simulink model "Power_Grid_Fault_Analysis_2016"  (R2016a)
settings: Solver=FixedStepAuto  SolverMode=SingleTasking  StartTime=0.0  StopTime=0.2  RelTol=1e-3
InitFcn:
  | basekV = 23;
  | baseMVA = 100;
  | 
  | % base impedance
  | baseZ = (basekV)^2/baseMVA;
  | 
  | % nominal frequency
  | freq = 50;
libraries: powerlib x64, powerlib_meascontrol x17
(part 4 of 4)

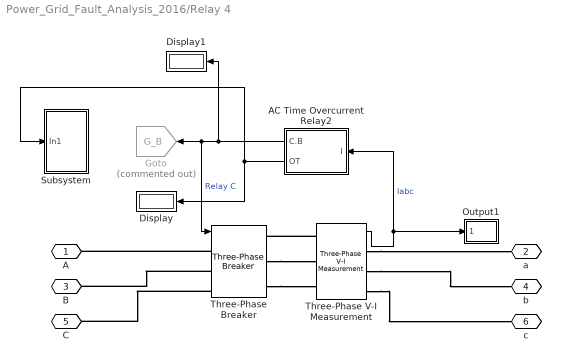
== system Power_Grid_Fault_Analysis_2016/Relay 4 ==
  AC Time Overcurrent Relay2 : Subsystem  mask(AC Time Overcurrent Relay Block){tcpopup=Definite Minimum Time, k=0, alpha=0.02, B=0, PS=100%, TMS=0.1, TDS=5, CTpri=300, CTsec=5, Freq=60, RMSInit=0}
      mask prompts: tcpopup "Trip Characteristic"; PS "Plug Setting (PS) / Low-set (I >)"; TMS "Time Multiplier Setting (TMS)"; TDS "Time Delay Setting (TDS) in sec"; CTpri "Current Transformer Primary (A)"; CTsec "Current Transformer Secondary (A)"; Freq "Fundamental frequency (Hz):"; RMSInit "Initial RMS value:"
      mask help:
      | AC Time Overcurrent Relay Block developed by Dr Rodney Tan
      | Version 1.0 (Jun 2016)
      |
      | AC Time Overcurrent Relay (ANSI/IEEE C37.2 device number 51) that operates when the current exceeds a predetermined value.
      |
      | This relay operates with either a Definite Minimum Time (DMT) or Inverse Definite Minimum Time (IDMT) characteristic.
      |
      | This relay support both IEC 60255 Standard and IEEE Standard C37.112-1996 IDMT trip characteristic.
      mask Help:
      | <b><u>Block Setting</u></b>
      | <b>Trip Characteristic</b>
      | Relay operation mode selection of Definite Minimum Time (DMT), IEC 60255 Standard or IEEE Standard C37.112-1996 Inverse Definite Minimum Time (IDMT).
      | 
      | <b>Plug-Setting(PS) / Low-set (I >)</b>
      | Specify relay pick-up current based on current transformer rating ranging from 25% to 200% with 25% step interval.
      | 
      | <b>Time Multiplier Setting (TMS)</b>
      | Specify time delay multiplier ranging from 0.05 to 1.0 for IDMT relay operation. This setting will be disabled DMT relay operation mode.
      | 
      | <b>Plot Curve Button</b>
      | Plot current Inverse Definite Minimum Time trip curve.
      | 
      | <b>Time Delay Setting (TDS)</b>
      | Specify time delay ranging from 0.05sec to 99sec for Definite Minimum Time relay operation. This setting will be disabled in IDMT relay operation mode.
      | 
      | <b>Current Transformer Primary (A)</b>
      | Specify current transformer primary in Ampere.
      | 
      | <b>Current Transformer Secondary (A)</b>
      | Specify current transformer secondary in Ampere.
      | 
      | <b>Fundamental Frequency (Hz)</b>
      | Specify the RMS current measurement fundamental frequency, in hertz, of the input signal.
      | 
      | <b>Initial RMS Value</b>
      | Specify the RMS current measurement initial RMS value of the output signal.
      | 
      | <b><u>Block Input Output</u></b>
      | <b>I</b>
      | Current input to the AC time overcurrent relay
      | 
      | <b>trip</b>
      | Trip control signal output (1-0), commonly connected to circuit breaker
      | 
      | <b>OT</b>
      | Relay operating time output
      mask TypeOptions tcpopup: Definite Minimum Time | IEC Standard Inverse | IEC Very Inverse | IEC Long Time Inverse | IEC Extremely Inverse | IEC Ultra Inverse | IEEE Moderately Inverse | IEEE Very Inverse | IEEE Extremely Inverse
      mask Callback tcpopup:
      | switch(get_param(gcb,'tcpopup'))
      |     case 'IEC Standard Inverse'
      |         set_param(gcb,'k','0.14');
      |         set_param(gcb,'alpha','0.02');
      |         set_param(gcb,'B','0');
      |         set_param(gcb,'MaskEnables',{'on','off','off','off',...
      |                   'on','on','off','on','on','on','on'});
      |     case 'IEC Very Inverse'
      |         set_param(gcb,'k','13.5');
      |         set_param(gcb,'alpha','1');
      |         set_param(gcb,'B','0');
      |         set_param(gcb,'MaskEnables',{'on','off','off','off',...
      |                   'on','on','off','on','on','on','on'});
      |     case 'IEC Long Time Inverse'
      |         set_param(gcb,'k','120');
      |         set_param(gcb,'alpha','1');
      |         set_param(gcb,'B','0');
      |         set_param(gcb,'MaskEnables',{'on','off','off','off',...
      |                   'on','on','off','on','on','on','on'});
      |     case 'IEC Extremely Inverse'
      |         set_param(gcb,'k','80');
      |         set_param(gcb,'alpha','2');
      |         set_param(gcb,'B','0');
      |         set_param(gcb,'MaskEnables',{'on','off','off','off',...
      |                   'on','on','off','on','on','on','on'});
      |     case 'IEC Ultra Inverse'
      |         set_param(gcb,'k','315.2');
      |         set_param(gcb,'alpha','2.5');
      |         set_param(gcb,'B','0');
      |         set_param(gcb,'MaskEnables',{'on','off','off','off',...
      |                   'on','on','off','on','on','on','on'});
      |     case 'IEEE Moderately Inverse'
      |         set_param(gcb,'k','0.0515');
      |         set_param(gcb,'alpha','0.02');
      |         set_param(gcb,'B','0.114');
      |         set_param(gcb,'MaskEnables',{'on','off','off','off',...
      |                   'on','on','off','on','on','on','on'});
      |     case 'IEEE Very Inverse'
      |         set_param(gcb,'k','19.61');
      |         set_param(gcb,'alpha','2');
      |         set_param(gcb,'B','0.491');
      |         set_param(gcb,'MaskEnables',{'on','off','off','off',...
      |                   'on','on','off','on','on','on','on'});
      |     case 'IEEE Extremely Inverse'
      |         set_param(gcb,'k','28.2');
      |         set_param(gcb,'alpha','2');
      |         set_param(gcb,'B','0.1217');
      |         set_param(gcb,'MaskEnables',{'on','off','off','off',...
      |                   'on','on','off','on','on','on','on'});
      |     otherwise
      |         set_param(gcb,'k','0');
      |         set_param(gcb,'MaskEnables',{'on','off','off','off',...
      |                   'on','off','on','on','on','on','on'});
      | end
      mask TypeOptions PS: 25% | 50% | 75% | 100% | 125% | 150% | 175% | 200%
      mask TypeOptions TMS: 0.05 | 0.1 | 0.15 | 0.2 | 0.25 | 0.3 | 0.35 | 0.4 | 0.45 | 0.5 | 0.55 | 0.6 | 0.65 | 0.7 | 0.75 | 0.8 | 0.85 | 0.9 | 0.95 | 1.0
      mask Callback TDS:
      | TDS = str2double(get_param(gcb,'TDS'));
      | if (TDS > 99)||(TDS < 0.05)||isnan(TDS)
      |     msgbox('TDS must be in the range of 0.05-99 sec',...
      |     'Invalid Value !','error');
      |     set_param(gcb,'TDS','0.1');
      | end
      mask TypeOptions Freq: Irms/Freq
      mask TypeOptions RMSInit: Irms/RMSInit
      mask DialogControl plotbutton Prompt: Plot Curve
      mask DialogControl plotbutton Callback:
      | % Plotting IDMT Curve
      | TMS = str2num(get_param(gcb,'TMS'));
      | k = str2num(get_param(gcb,'k'));
      | alpha = str2num(get_param(gcb,'alpha'));
      | B = str2num(get_param(gcb,'B'));
      | I = 1:20;
      | td = ((k./((I.^alpha)-1))+B)*TMS;
      | loglog(td);
      | set(gcf, 'Position', [200 150 300 500]);
      | switch(get_param(gcb,'tcpopup'))
      |     case 'IEC Standard Inverse'
      |         title('IEC Standard Inverse');
      |         set(gca, 'YTick', (1:10));
      |         ylim([0.1 10]);
      |     case 'IEC Very Inverse'
      |         title('IEC Very Inverse');
      |         set(gca, 'YTick', (1:2:15));
      |         ylim([0.01 15]);
      |     case 'IEC Long Time Inverse'
      |         title('IEC Long Time Inverse');
      |         set(gca, 'YTick', (0:20:120));
      |         ylim([0.1 120]);
      |     case 'IEC Extremely Inverse'
      |         title('IEC Extremely Inverse');
      |         set(gca, 'YTick', (0:5:30));
      |         ylim([0.01 30]);
      |     case 'IEC Ultra Inverse'
      |         title('IEC Ultra Inverse');
      |         set(gca, 'YTick', (0:20:100));
      |         ylim([0.01 100]);
      |     case 'IEEE Moderately Inverse'
      |         title('IEEE Moderately Inverse');
      |         set(gca, 'YTick', (1:5));
      |         ylim([0.01 5]);
      |     case 'IEEE Very Inverse'
      |         title('IEEE Very Inverse');
      |         set(gca, 'YTick', (1:10));
      |         ylim([0.01 10]);
      |     case 'IEEE Extremely Inverse'
      |         title('IEEE Extremely Inverse');
      |         set(gca, 'YTick', (1:10));
      |         ylim([0.01 10]);
      | end
      | 
      | set(gca, 'XTick', [1:10 20]);
      | xlim([1 30]);
      | xlabel('Current (Multiples of Plug Setting)');
      | ylabel('Operating Time (sec)');
      | grid on;
      mask DialogControl RMS Prompt: RMS Current Measurement
      mask Display:
      | disp('(51)');
      | port_label('input', 1, 'I');
      | port_label('output', 1, 'trip');
      | port_label('output', 2, 'OT');
  Display : Display
  Display1 : Display
  Goto : Goto  Commented=on  GotoTag=G_B  TagVisibility=global
  Output1 : Subsystem
  Subsystem : Subsystem
  Three-Phase V-I Measurement : powerlib/Measurements/Three-Phase V-I Measurement  VoltageMeasurement=no  SetLabelV=off  LabelV=Vabc  Vpu=off  VpuLL=off  CurrentMeasurement=yes  SetLabelI=off  LabelI=Iabc  Ipu=off  Pbase=100e6  Vbase=500e3  OutputType=Complex  PhasorSimulation=off  PSBequivalent=0
  Three-Phase Breaker : powerlib/Elements/Three-Phase Breaker  InitialState=closed  SwitchA=on  SwitchB=on  SwitchC=on  SwitchTimes="[1/60  5/60]"  External=on  BreakerResistance=0.001  SnubberResistance=1e6  SnubberCapacitance=inf  Measurements=None
  A : PMIOPort  Side=Left
  a : PMIOPort  Port=2  Side=Right
  B : PMIOPort  Port=3  Side=Left
  b : PMIOPort  Port=4  Side=Right
  C : PMIOPort  Port=5  Side=Left
  c : PMIOPort  Port=6  Side=Right
  wires:
  Three-Phase V-I Measurement/1 -> Output1/1(Signal), AC Time Overcurrent Relay2/1(I)  "Iabc"
  AC Time Overcurrent Relay2/2(OT) -> Subsystem/1(In1), Display/1
  AC Time Overcurrent Relay2/1(C.B) -> Display1/1, Goto/1, Three-Phase Breaker/1  "Relay C"
  connections:
  Three-Phase Breaker/RConn2 -- Three-Phase V-I Measurement/LConn2
  Three-Phase V-I Measurement/RConn2 -- b/RConn1
  Three-Phase V-I Measurement/LConn1 -- Three-Phase Breaker/RConn1
  Three-Phase Breaker/LConn2 -- B/RConn1
  Three-Phase V-I Measurement/RConn1 -- a/RConn1
  Three-Phase Breaker/RConn3 -- Three-Phase V-I Measurement/LConn3
  Three-Phase Breaker/LConn3 -- C/RConn1
  Three-Phase V-I Measurement/RConn3 -- c/RConn1
  Three-Phase Breaker/LConn1 -- A/RConn1

== system Power_Grid_Fault_Analysis_2016/Toggle Switch ==

== system Power_Grid_Fault_Analysis_2016/Toggle Switch1 ==

== system Power_Grid_Fault_Analysis_2016/Toggle Switch2 ==

== system Power_Grid_Fault_Analysis_2016/Toggle Switch3 ==

== system Power_Grid_Fault_Analysis_2016/Toggle Switch4 ==

== system Power_Grid_Fault_Analysis_2016/Bus_10/VI Recorder7 ==
  Vrec : Inport
  Irec : Inport  Port=2
  tag scope: I8to10=global, V8to10=global
  wires:
  Vrec/1 -> [V8to10]
  Irec/1 -> [I8to10]

== system Power_Grid_Fault_Analysis_2016/Bus_11/VI Recorder7 ==
  Vrec : Inport
  Irec : Inport  Port=2
  tag scope: I9to11=global, V9to11=global
  wires:
  Vrec/1 -> [V9to11]
  Irec/1 -> [I9to11]

== system Power_Grid_Fault_Analysis_2016/Bus_12/VI Recorder7 ==
  Vrec : Inport
  Irec : Inport  Port=2
  tag scope: I9to12=global, V9to12=global
  wires:
  Vrec/1 -> [V9to12]
  Irec/1 -> [I9to12]

== system Power_Grid_Fault_Analysis_2016/Bus_13/VI Recorder7 ==
  Vrec : Inport
  Irec : Inport  Port=2
  tag scope: I3to13=global, V3to13=global
  wires:
  Vrec/1 -> [V3to13]
  Irec/1 -> [I3to13]

== system Power_Grid_Fault_Analysis_2016/Bus_14/VI Recorder7 ==
  Vrec : Inport
  Irec : Inport  Port=2
  tag scope: I13to14=global, V13to14=global
  wires:
  Vrec/1 -> [V13to14]
  Irec/1 -> [I13to14]

== system Power_Grid_Fault_Analysis_2016/Bus_15/VI Recorder7 ==
  Vrec : Inport
  Irec : Inport  Port=2
  tag scope: I13to15=global, V13to15=global
  wires:
  Vrec/1 -> [V13to15]
  Irec/1 -> [I13to15]

== system Power_Grid_Fault_Analysis_2016/Bus_16/VI Recorder7 ==
  Vrec : Inport
  Irec : Inport  Port=2
  tag scope: I15to16=global, V15to16=global
  wires:
  Vrec/1 -> [V15to16]
  Irec/1 -> [I15to16]

== system Power_Grid_Fault_Analysis_2016/Bus_4/VI Recorder7 ==
  Vrec : Inport
  Irec : Inport  Port=2
  tag scope: I1to4=global, V1to4=global
  wires:
  Vrec/1 -> [V1to4]
  Irec/1 -> [I1to4]

== system Power_Grid_Fault_Analysis_2016/Bus_5/VI Recorder7 ==
  Vrec : Inport
  Irec : Inport  Port=2
  tag scope: I4to5=global, V4to5=global
  wires:
  Vrec/1 -> [V4to5]
  Irec/1 -> [I4to5]

== system Power_Grid_Fault_Analysis_2016/Bus_6/VI Recorder7 ==
  Vrec : Inport
  Irec : Inport  Port=2
  tag scope: I4to6=global, V4to6=global
  wires:
  Vrec/1 -> [V4to6]
  Irec/1 -> [I4to6]

== system Power_Grid_Fault_Analysis_2016/Bus_7/VI Recorder7 ==
  Vrec : Inport
  Irec : Inport  Port=2
  tag scope: I6to7=global, V6to7=global
  wires:
  Vrec/1 -> [V6to7]
  Irec/1 -> [I6to7]

== system Power_Grid_Fault_Analysis_2016/Bus_8/VI Recorder7 ==
  Vrec : Inport
  Irec : Inport  Port=2
  tag scope: I2to8=global, V2to8=global
  wires:
  Vrec/1 -> [V2to8]
  Irec/1 -> [I2to8]

== system Power_Grid_Fault_Analysis_2016/Bus_9/VI Recorder7 ==
  Vrec : Inport
  Irec : Inport  Port=2
  tag scope: I8to9=global, V8to9=global
  wires:
  Vrec/1 -> [V8to9]
  Irec/1 -> [I8to9]

== system Power_Grid_Fault_Analysis_2016/For Zone 1/If Action Subsystem ==
  Input : Inport
  Input1 : Inport  Port=2
  Input2 : Inport  Port=3
  Action Port : ActionPort
  Out1 : Outport
  Out2 : Outport  Port=2
  Out3 : Outport  Port=3
  wires:
  Input/1 -> Out1/1
  Input1/1 -> Out2/1
  Input2/1 -> Out3/1

== system Power_Grid_Fault_Analysis_2016/For Zone 1/If Action Subsystem1 ==
  Input : Inport
  Input1 : Inport  Port=2
  Input2 : Inport  Port=3
  Action Port : ActionPort
  Out1 : Outport
  Out2 : Outport  Port=2
  Out3 : Outport  Port=3
  wires:
  Input/1 -> Out1/1
  Input1/1 -> Out2/1
  Input2/1 -> Out3/1

== system Power_Grid_Fault_Analysis_2016/For Zone 1/If Action Subsystem2 ==
  Input : Inport
  Input1 : Inport  Port=2
  Input2 : Inport  Port=3
  Action Port : ActionPort
  Out1 : Outport
  Out2 : Outport  Port=2
  Out3 : Outport  Port=3
  wires:
  Input/1 -> Out1/1
  Input1/1 -> Out2/1
  Input2/1 -> Out3/1

== system Power_Grid_Fault_Analysis_2016/For Zone 1/If Action Subsystem3 ==
  Input : Inport
  Input1 : Inport  Port=2
  Input2 : Inport  Port=3
  Action Port : ActionPort
  Out1 : Outport
  Out2 : Outport  Port=2
  Out3 : Outport  Port=3
  wires:
  Input/1 -> Out1/1
  Input1/1 -> Out2/1
  Input2/1 -> Out3/1

== system Power_Grid_Fault_Analysis_2016/For Zone 1/If Action Subsystem4 ==
  Input : Inport
  Input1 : Inport  Port=2
  Input2 : Inport  Port=3
  Action Port : ActionPort
  Out1 : Outport
  Out2 : Outport  Port=2
  Out3 : Outport  Port=3
  wires:
  Input/1 -> Out1/1
  Input1/1 -> Out2/1
  Input2/1 -> Out3/1

== system Power_Grid_Fault_Analysis_2016/For Zone 1/If Action Subsystem5 ==
  Input : Inport
  Input1 : Inport  Port=2
  Input2 : Inport  Port=3
  Action Port : ActionPort
  Out1 : Outport
  Out2 : Outport  Port=2
  Out3 : Outport  Port=3
  wires:
  Input/1 -> Out1/1
  Input1/1 -> Out2/1
  Input2/1 -> Out3/1

== system Power_Grid_Fault_Analysis_2016/For Zone 1/If Action Subsystem6 ==
  Input : Inport
  Input1 : Inport  Port=2
  Input2 : Inport  Port=3
  Action Port : ActionPort
  Out1 : Outport
  Out2 : Outport  Port=2
  Out3 : Outport  Port=3
  wires:
  Input/1 -> Out1/1
  Input1/1 -> Out2/1
  Input2/1 -> Out3/1

== system Power_Grid_Fault_Analysis_2016/For Zone 1/Subsystem1 ==
  In1 : Inport
  In2 : Inport  Port=2
  Display2 : Display
      settings: Decimation=2
  Divide4 : Product  Inputs=**  SaturateOnIntegerOverflow=on  RndMeth=Zero
  Output : Outport
  wires:
  Divide4/1 -> Display2/1, Output/1
  In1/1 -> Divide4/1
  In2/1 -> Divide4/2

== system Power_Grid_Fault_Analysis_2016/For Zone 1/Subsystem2 ==
  In1 : Inport
  In2 : Inport  Port=2
  Display2 : Display
      settings: Decimation=2
  Divide4 : Product  Inputs=**  SaturateOnIntegerOverflow=on  RndMeth=Zero
  Output : Outport
  wires:
  In2/1 -> Divide4/2
  In1/1 -> Divide4/1
  Divide4/1 -> Output/1, Display2/1

== system Power_Grid_Fault_Analysis_2016/For Zone 1/Subsystem3 ==
  In1 : Inport
  In2 : Inport  Port=2
  Display2 : Display
      settings: Decimation=2
  Divide4 : Product  Inputs=**  SaturateOnIntegerOverflow=on  RndMeth=Zero
  Output : Outport
  wires:
  In2/1 -> Divide4/2
  In1/1 -> Divide4/1
  Divide4/1 -> Output/1, Display2/1

== system Power_Grid_Fault_Analysis_2016/For Zone 1/Subsystem4 ==
  In1 : Inport
  In2 : Inport  Port=2
  Display2 : Display
      settings: Decimation=2
  Divide4 : Product  Inputs=**  SaturateOnIntegerOverflow=on  RndMeth=Zero
  Output : Outport
  wires:
  Divide4/1 -> Display2/1, Output/1
  In1/1 -> Divide4/1
  In2/1 -> Divide4/2

== system Power_Grid_Fault_Analysis_2016/For Zone 1/Subsystem5 ==
  In1 : Inport
  In2 : Inport  Port=2
  Display2 : Display
      settings: Decimation=2
  Divide4 : Product  Inputs=**  SaturateOnIntegerOverflow=on  RndMeth=Zero
  Output : Outport
  wires:
  In2/1 -> Divide4/2
  In1/1 -> Divide4/1
  Divide4/1 -> Output/1, Display2/1

== system Power_Grid_Fault_Analysis_2016/For Zone 1/Subsystem6 ==
  In1 : Inport
  In2 : Inport  Port=2
  Display2 : Display
      settings: Decimation=2
  Divide4 : Product  Inputs=**  SaturateOnIntegerOverflow=on  RndMeth=Zero
  Output : Outport
  wires:
  Divide4/1 -> Display2/1, Output/1
  In1/1 -> Divide4/1
  In2/1 -> Divide4/2

== system Power_Grid_Fault_Analysis_2016/For Zone 1/Subsystem7 ==
  In1 : Inport
  In2 : Inport  Port=2
  Display2 : Display
      settings: Decimation=2
  Divide4 : Product  Inputs=**  SaturateOnIntegerOverflow=on  RndMeth=Zero
  Output : Outport
  wires:
  In2/1 -> Divide4/2
  In1/1 -> Divide4/1
  Divide4/1 -> Output/1, Display2/1

== system Power_Grid_Fault_Analysis_2016/For Zone 2/If Action Subsystem ==
  Input : Inport
  Input1 : Inport  Port=2
  Input2 : Inport  Port=3
  Action Port : ActionPort
  Out1 : Outport
  Out2 : Outport  Port=2
  Out3 : Outport  Port=3
  wires:
  Input/1 -> Out1/1
  Input1/1 -> Out2/1
  Input2/1 -> Out3/1

== system Power_Grid_Fault_Analysis_2016/For Zone 2/If Action Subsystem1 ==
  Input : Inport
  Input1 : Inport  Port=2
  Input2 : Inport  Port=3
  Action Port : ActionPort
  Out1 : Outport
  Out2 : Outport  Port=2
  Out3 : Outport  Port=3
  wires:
  Input/1 -> Out1/1
  Input1/1 -> Out2/1
  Input2/1 -> Out3/1

== system Power_Grid_Fault_Analysis_2016/For Zone 2/If Action Subsystem2 ==
  Input : Inport
  Input1 : Inport  Port=2
  Input2 : Inport  Port=3
  Action Port : ActionPort
  Out1 : Outport
  Out2 : Outport  Port=2
  Out3 : Outport  Port=3
  wires:
  Input/1 -> Out1/1
  Input1/1 -> Out2/1
  Input2/1 -> Out3/1

== system Power_Grid_Fault_Analysis_2016/For Zone 2/If Action Subsystem3 ==
  Input : Inport
  Input1 : Inport  Port=2
  Input2 : Inport  Port=3
  Action Port : ActionPort
  Out1 : Outport
  Out2 : Outport  Port=2
  Out3 : Outport  Port=3
  wires:
  Input/1 -> Out1/1
  Input1/1 -> Out2/1
  Input2/1 -> Out3/1

== system Power_Grid_Fault_Analysis_2016/For Zone 2/If Action Subsystem4 ==
  Input : Inport
  Input1 : Inport  Port=2
  Input2 : Inport  Port=3
  Action Port : ActionPort
  Out1 : Outport
  Out2 : Outport  Port=2
  Out3 : Outport  Port=3
  wires:
  Input/1 -> Out1/1
  Input1/1 -> Out2/1
  Input2/1 -> Out3/1

== system Power_Grid_Fault_Analysis_2016/For Zone 2/If Action Subsystem5 ==
  Input : Inport
  Input1 : Inport  Port=2
  Input2 : Inport  Port=3
  Action Port : ActionPort
  Out1 : Outport
  Out2 : Outport  Port=2
  Out3 : Outport  Port=3
  wires:
  Input/1 -> Out1/1
  Input1/1 -> Out2/1
  Input2/1 -> Out3/1

== system Power_Grid_Fault_Analysis_2016/For Zone 2/If Action Subsystem6 ==
  Input : Inport
  Input1 : Inport  Port=2
  Input2 : Inport  Port=3
  Action Port : ActionPort
  Out1 : Outport
  Out2 : Outport  Port=2
  Out3 : Outport  Port=3
  wires:
  Input/1 -> Out1/1
  Input1/1 -> Out2/1
  Input2/1 -> Out3/1

== system Power_Grid_Fault_Analysis_2016/For Zone 2/Subsystem1 ==
  In1 : Inport
  In2 : Inport  Port=2
  Display2 : Display
      settings: Decimation=2
  Divide4 : Product  Inputs=**  SaturateOnIntegerOverflow=on  RndMeth=Zero
  Output : Outport
  wires:
  Divide4/1 -> Display2/1, Output/1
  In1/1 -> Divide4/1
  In2/1 -> Divide4/2

== system Power_Grid_Fault_Analysis_2016/For Zone 2/Subsystem2 ==
  In1 : Inport
  In2 : Inport  Port=2
  Display2 : Display
      settings: Decimation=2
  Divide4 : Product  Inputs=**  SaturateOnIntegerOverflow=on  RndMeth=Zero
  Output : Outport
  wires:
  In2/1 -> Divide4/2
  In1/1 -> Divide4/1
  Divide4/1 -> Output/1, Display2/1

== system Power_Grid_Fault_Analysis_2016/For Zone 2/Subsystem3 ==
  In1 : Inport
  In2 : Inport  Port=2
  Display2 : Display
      settings: Decimation=2
  Divide4 : Product  Inputs=**  SaturateOnIntegerOverflow=on  RndMeth=Zero
  Output : Outport
  wires:
  In2/1 -> Divide4/2
  In1/1 -> Divide4/1
  Divide4/1 -> Output/1, Display2/1

== system Power_Grid_Fault_Analysis_2016/For Zone 2/Subsystem4 ==
  In1 : Inport
  In2 : Inport  Port=2
  Display2 : Display
      settings: Decimation=2
  Divide4 : Product  Inputs=**  SaturateOnIntegerOverflow=on  RndMeth=Zero
  Output : Outport
  wires:
  Divide4/1 -> Display2/1, Output/1
  In1/1 -> Divide4/1
  In2/1 -> Divide4/2

== system Power_Grid_Fault_Analysis_2016/For Zone 2/Subsystem5 ==
  In1 : Inport
  In2 : Inport  Port=2
  Display2 : Display
      settings: Decimation=2
  Divide4 : Product  Inputs=**  SaturateOnIntegerOverflow=on  RndMeth=Zero
  Output : Outport
  wires:
  In2/1 -> Divide4/2
  In1/1 -> Divide4/1
  Divide4/1 -> Output/1, Display2/1

== system Power_Grid_Fault_Analysis_2016/For Zone 2/Subsystem6 ==
  In1 : Inport
  In2 : Inport  Port=2
  Display2 : Display
      settings: Decimation=2
  Divide4 : Product  Inputs=**  SaturateOnIntegerOverflow=on  RndMeth=Zero
  Output : Outport
  wires:
  Divide4/1 -> Display2/1, Output/1
  In1/1 -> Divide4/1
  In2/1 -> Divide4/2

== system Power_Grid_Fault_Analysis_2016/For Zone 2/Subsystem7 ==
  In1 : Inport
  In2 : Inport  Port=2
  Display2 : Display
      settings: Decimation=2
  Divide4 : Product  Inputs=**  SaturateOnIntegerOverflow=on  RndMeth=Zero
  Output : Outport
  wires:
  In2/1 -> Divide4/2
  In1/1 -> Divide4/1
  Divide4/1 -> Output/1, Display2/1

== system Power_Grid_Fault_Analysis_2016/For Zone 3/If Action Subsystem ==
  Input : Inport
  Input1 : Inport  Port=2
  Input2 : Inport  Port=3
  Action Port : ActionPort
  Out1 : Outport
  Out2 : Outport  Port=2
  Out3 : Outport  Port=3
  wires:
  Input/1 -> Out1/1
  Input1/1 -> Out2/1
  Input2/1 -> Out3/1

== system Power_Grid_Fault_Analysis_2016/For Zone 3/If Action Subsystem1 ==
  Input : Inport
  Input1 : Inport  Port=2
  Input2 : Inport  Port=3
  Action Port : ActionPort
  Out1 : Outport
  Out2 : Outport  Port=2
  Out3 : Outport  Port=3
  wires:
  Input/1 -> Out1/1
  Input1/1 -> Out2/1
  Input2/1 -> Out3/1

== system Power_Grid_Fault_Analysis_2016/For Zone 3/If Action Subsystem2 ==
  Input : Inport
  Input1 : Inport  Port=2
  Input2 : Inport  Port=3
  Action Port : ActionPort
  Out1 : Outport
  Out2 : Outport  Port=2
  Out3 : Outport  Port=3
  wires:
  Input/1 -> Out1/1
  Input1/1 -> Out2/1
  Input2/1 -> Out3/1

== system Power_Grid_Fault_Analysis_2016/For Zone 3/If Action Subsystem3 ==
  Input : Inport
  Input1 : Inport  Port=2
  Input2 : Inport  Port=3
  Action Port : ActionPort
  Out1 : Outport
  Out2 : Outport  Port=2
  Out3 : Outport  Port=3
  wires:
  Input/1 -> Out1/1
  Input1/1 -> Out2/1
  Input2/1 -> Out3/1

== system Power_Grid_Fault_Analysis_2016/For Zone 3/If Action Subsystem4 ==
  Input : Inport
  Input1 : Inport  Port=2
  Input2 : Inport  Port=3
  Action Port : ActionPort
  Out1 : Outport
  Out2 : Outport  Port=2
  Out3 : Outport  Port=3
  wires:
  Input/1 -> Out1/1
  Input1/1 -> Out2/1
  Input2/1 -> Out3/1

== system Power_Grid_Fault_Analysis_2016/For Zone 3/If Action Subsystem5 ==
  Input : Inport
  Input1 : Inport  Port=2
  Input2 : Inport  Port=3
  Action Port : ActionPort
  Out1 : Outport
  Out2 : Outport  Port=2
  Out3 : Outport  Port=3
  wires:
  Input/1 -> Out1/1
  Input1/1 -> Out2/1
  Input2/1 -> Out3/1

== system Power_Grid_Fault_Analysis_2016/For Zone 3/If Action Subsystem6 ==
  Input : Inport
  Input1 : Inport  Port=2
  Input2 : Inport  Port=3
  Action Port : ActionPort
  Out1 : Outport
  Out2 : Outport  Port=2
  Out3 : Outport  Port=3
  wires:
  Input/1 -> Out1/1
  Input1/1 -> Out2/1
  Input2/1 -> Out3/1

== system Power_Grid_Fault_Analysis_2016/For Zone 3/Subsystem1 ==
  In1 : Inport
  In2 : Inport  Port=2
  Display2 : Display
      settings: Decimation=2
  Divide4 : Product  Inputs=**  SaturateOnIntegerOverflow=on  RndMeth=Zero
  Output : Outport
  wires:
  Divide4/1 -> Display2/1, Output/1
  In1/1 -> Divide4/1
  In2/1 -> Divide4/2

== system Power_Grid_Fault_Analysis_2016/For Zone 3/Subsystem2 ==
  In1 : Inport
  In2 : Inport  Port=2
  Display2 : Display
      settings: Decimation=2
  Divide4 : Product  Inputs=**  SaturateOnIntegerOverflow=on  RndMeth=Zero
  Output : Outport
  wires:
  In2/1 -> Divide4/2
  In1/1 -> Divide4/1
  Divide4/1 -> Output/1, Display2/1

== system Power_Grid_Fault_Analysis_2016/For Zone 3/Subsystem3 ==
  In1 : Inport
  In2 : Inport  Port=2
  Display2 : Display
      settings: Decimation=2
  Divide4 : Product  Inputs=**  SaturateOnIntegerOverflow=on  RndMeth=Zero
  Output : Outport
  wires:
  In2/1 -> Divide4/2
  In1/1 -> Divide4/1
  Divide4/1 -> Output/1, Display2/1

== system Power_Grid_Fault_Analysis_2016/For Zone 3/Subsystem4 ==
  In1 : Inport
  In2 : Inport  Port=2
  Display2 : Display
      settings: Decimation=2
  Divide4 : Product  Inputs=**  SaturateOnIntegerOverflow=on  RndMeth=Zero
  Output : Outport
  wires:
  Divide4/1 -> Display2/1, Output/1
  In1/1 -> Divide4/1
  In2/1 -> Divide4/2

== system Power_Grid_Fault_Analysis_2016/For Zone 3/Subsystem5 ==
  In1 : Inport
  In2 : Inport  Port=2
  Display2 : Display
      settings: Decimation=2
  Divide4 : Product  Inputs=**  SaturateOnIntegerOverflow=on  RndMeth=Zero
  Output : Outport
  wires:
  In2/1 -> Divide4/2
  In1/1 -> Divide4/1
  Divide4/1 -> Output/1, Display2/1

== system Power_Grid_Fault_Analysis_2016/For Zone 3/Subsystem6 ==
  In1 : Inport
  In2 : Inport  Port=2
  Display2 : Display
      settings: Decimation=2
  Divide4 : Product  Inputs=**  SaturateOnIntegerOverflow=on  RndMeth=Zero
  Output : Outport
  wires:
  Divide4/1 -> Display2/1, Output/1
  In1/1 -> Divide4/1
  In2/1 -> Divide4/2

== system Power_Grid_Fault_Analysis_2016/For Zone 3/Subsystem7 ==
  In1 : Inport
  In2 : Inport  Port=2
  Display2 : Display
      settings: Decimation=2
  Divide4 : Product  Inputs=**  SaturateOnIntegerOverflow=on  RndMeth=Zero
  Output : Outport
  wires:
  In2/1 -> Divide4/2
  In1/1 -> Divide4/1
  Divide4/1 -> Output/1, Display2/1

== system Power_Grid_Fault_Analysis_2016/For Zone 4/If Action Subsystem ==
  Input : Inport
  Input1 : Inport  Port=2
  Input2 : Inport  Port=3
  Action Port : ActionPort
  Out1 : Outport
  Out2 : Outport  Port=2
  Out3 : Outport  Port=3
  wires:
  Input/1 -> Out1/1
  Input1/1 -> Out2/1
  Input2/1 -> Out3/1

== system Power_Grid_Fault_Analysis_2016/For Zone 4/If Action Subsystem1 ==
  Input : Inport
  Input1 : Inport  Port=2
  Input2 : Inport  Port=3
  Action Port : ActionPort
  Out1 : Outport
  Out2 : Outport  Port=2
  Out3 : Outport  Port=3
  wires:
  Input/1 -> Out1/1
  Input1/1 -> Out2/1
  Input2/1 -> Out3/1

== system Power_Grid_Fault_Analysis_2016/For Zone 4/If Action Subsystem2 ==
  Input : Inport
  Input1 : Inport  Port=2
  Input2 : Inport  Port=3
  Action Port : ActionPort
  Out1 : Outport
  Out2 : Outport  Port=2
  Out3 : Outport  Port=3
  wires:
  Input/1 -> Out1/1
  Input1/1 -> Out2/1
  Input2/1 -> Out3/1

== system Power_Grid_Fault_Analysis_2016/For Zone 4/If Action Subsystem3 ==
  Input : Inport
  Input1 : Inport  Port=2
  Input2 : Inport  Port=3
  Action Port : ActionPort
  Out1 : Outport
  Out2 : Outport  Port=2
  Out3 : Outport  Port=3
  wires:
  Input/1 -> Out1/1
  Input1/1 -> Out2/1
  Input2/1 -> Out3/1

== system Power_Grid_Fault_Analysis_2016/For Zone 4/If Action Subsystem4 ==
  Input : Inport
  Input1 : Inport  Port=2
  Input2 : Inport  Port=3
  Action Port : ActionPort
  Out1 : Outport
  Out2 : Outport  Port=2
  Out3 : Outport  Port=3
  wires:
  Input/1 -> Out1/1
  Input1/1 -> Out2/1
  Input2/1 -> Out3/1

== system Power_Grid_Fault_Analysis_2016/For Zone 4/If Action Subsystem5 ==
  Input : Inport
  Input1 : Inport  Port=2
  Input2 : Inport  Port=3
  Action Port : ActionPort
  Out1 : Outport
  Out2 : Outport  Port=2
  Out3 : Outport  Port=3
  wires:
  Input/1 -> Out1/1
  Input1/1 -> Out2/1
  Input2/1 -> Out3/1

== system Power_Grid_Fault_Analysis_2016/For Zone 4/If Action Subsystem6 ==
  Input : Inport
  Input1 : Inport  Port=2
  Input2 : Inport  Port=3
  Action Port : ActionPort
  Out1 : Outport
  Out2 : Outport  Port=2
  Out3 : Outport  Port=3
  wires:
  Input/1 -> Out1/1
  Input1/1 -> Out2/1
  Input2/1 -> Out3/1

== system Power_Grid_Fault_Analysis_2016/For Zone 4/Subsystem1 ==
  In1 : Inport
  In2 : Inport  Port=2
  Display2 : Display
      settings: Decimation=2
  Divide4 : Product  Inputs=**  SaturateOnIntegerOverflow=on  RndMeth=Zero
  Output : Outport
  wires:
  Divide4/1 -> Display2/1, Output/1
  In1/1 -> Divide4/1
  In2/1 -> Divide4/2

== system Power_Grid_Fault_Analysis_2016/For Zone 4/Subsystem2 ==
  In1 : Inport
  In2 : Inport  Port=2
  Display2 : Display
      settings: Decimation=2
  Divide4 : Product  Inputs=**  SaturateOnIntegerOverflow=on  RndMeth=Zero
  Output : Outport
  wires:
  In2/1 -> Divide4/2
  In1/1 -> Divide4/1
  Divide4/1 -> Output/1, Display2/1

== system Power_Grid_Fault_Analysis_2016/For Zone 4/Subsystem3 ==
  In1 : Inport
  In2 : Inport  Port=2
  Display2 : Display
      settings: Decimation=2
  Divide4 : Product  Inputs=**  SaturateOnIntegerOverflow=on  RndMeth=Zero
  Output : Outport
  wires:
  In2/1 -> Divide4/2
  In1/1 -> Divide4/1
  Divide4/1 -> Output/1, Display2/1

== system Power_Grid_Fault_Analysis_2016/For Zone 4/Subsystem4 ==
  In1 : Inport
  In2 : Inport  Port=2
  Display2 : Display
      settings: Decimation=2
  Divide4 : Product  Inputs=**  SaturateOnIntegerOverflow=on  RndMeth=Zero
  Output : Outport
  wires:
  Divide4/1 -> Display2/1, Output/1
  In1/1 -> Divide4/1
  In2/1 -> Divide4/2

== system Power_Grid_Fault_Analysis_2016/For Zone 4/Subsystem5 ==
  In1 : Inport
  In2 : Inport  Port=2
  Display2 : Display
      settings: Decimation=2
  Divide4 : Product  Inputs=**  SaturateOnIntegerOverflow=on  RndMeth=Zero
  Output : Outport
  wires:
  In2/1 -> Divide4/2
  In1/1 -> Divide4/1
  Divide4/1 -> Output/1, Display2/1

== system Power_Grid_Fault_Analysis_2016/For Zone 4/Subsystem6 ==
  In1 : Inport
  In2 : Inport  Port=2
  Display2 : Display
      settings: Decimation=2
  Divide4 : Product  Inputs=**  SaturateOnIntegerOverflow=on  RndMeth=Zero
  Output : Outport
  wires:
  Divide4/1 -> Display2/1, Output/1
  In1/1 -> Divide4/1
  In2/1 -> Divide4/2

== system Power_Grid_Fault_Analysis_2016/For Zone 4/Subsystem7 ==
  In1 : Inport
  In2 : Inport  Port=2
  Display2 : Display
      settings: Decimation=2
  Divide4 : Product  Inputs=**  SaturateOnIntegerOverflow=on  RndMeth=Zero
  Output : Outport
  wires:
  In2/1 -> Divide4/2
  In1/1 -> Divide4/1
  Divide4/1 -> Output/1, Display2/1

== system Power_Grid_Fault_Analysis_2016/For Zone 5/If Action Subsystem ==
  Input : Inport
  Input1 : Inport  Port=2
  Input2 : Inport  Port=3
  Action Port : ActionPort
  Out1 : Outport
  Out2 : Outport  Port=2
  Out3 : Outport  Port=3
  wires:
  Input/1 -> Out1/1
  Input1/1 -> Out2/1
  Input2/1 -> Out3/1

== system Power_Grid_Fault_Analysis_2016/For Zone 5/If Action Subsystem1 ==
  Input : Inport
  Input1 : Inport  Port=2
  Input2 : Inport  Port=3
  Action Port : ActionPort
  Out1 : Outport
  Out2 : Outport  Port=2
  Out3 : Outport  Port=3
  wires:
  Input/1 -> Out1/1
  Input1/1 -> Out2/1
  Input2/1 -> Out3/1

== system Power_Grid_Fault_Analysis_2016/For Zone 5/If Action Subsystem2 ==
  Input : Inport
  Input1 : Inport  Port=2
  Input2 : Inport  Port=3
  Action Port : ActionPort
  Out1 : Outport
  Out2 : Outport  Port=2
  Out3 : Outport  Port=3
  wires:
  Input/1 -> Out1/1
  Input1/1 -> Out2/1
  Input2/1 -> Out3/1

== system Power_Grid_Fault_Analysis_2016/For Zone 5/If Action Subsystem3 ==
  Input : Inport
  Input1 : Inport  Port=2
  Input2 : Inport  Port=3
  Action Port : ActionPort
  Out1 : Outport
  Out2 : Outport  Port=2
  Out3 : Outport  Port=3
  wires:
  Input/1 -> Out1/1
  Input1/1 -> Out2/1
  Input2/1 -> Out3/1

== system Power_Grid_Fault_Analysis_2016/For Zone 5/If Action Subsystem4 ==
  Input : Inport
  Input1 : Inport  Port=2
  Input2 : Inport  Port=3
  Action Port : ActionPort
  Out1 : Outport
  Out2 : Outport  Port=2
  Out3 : Outport  Port=3
  wires:
  Input/1 -> Out1/1
  Input1/1 -> Out2/1
  Input2/1 -> Out3/1

== system Power_Grid_Fault_Analysis_2016/For Zone 5/If Action Subsystem5 ==
  Input : Inport
  Input1 : Inport  Port=2
  Input2 : Inport  Port=3
  Action Port : ActionPort
  Out1 : Outport
  Out2 : Outport  Port=2
  Out3 : Outport  Port=3
  wires:
  Input/1 -> Out1/1
  Input1/1 -> Out2/1
  Input2/1 -> Out3/1

== system Power_Grid_Fault_Analysis_2016/For Zone 5/If Action Subsystem6 ==
  Input : Inport
  Input1 : Inport  Port=2
  Input2 : Inport  Port=3
  Action Port : ActionPort
  Out1 : Outport
  Out2 : Outport  Port=2
  Out3 : Outport  Port=3
  wires:
  Input/1 -> Out1/1
  Input1/1 -> Out2/1
  Input2/1 -> Out3/1

== system Power_Grid_Fault_Analysis_2016/For Zone 5/Subsystem1 ==
  In1 : Inport
  In2 : Inport  Port=2
  Display2 : Display
      settings: Decimation=2
  Divide4 : Product  Inputs=**  SaturateOnIntegerOverflow=on  RndMeth=Zero
  Output : Outport
  wires:
  Divide4/1 -> Display2/1, Output/1
  In1/1 -> Divide4/1
  In2/1 -> Divide4/2

== system Power_Grid_Fault_Analysis_2016/For Zone 5/Subsystem2 ==
  In1 : Inport
  In2 : Inport  Port=2
  Display2 : Display
      settings: Decimation=2
  Divide4 : Product  Inputs=**  SaturateOnIntegerOverflow=on  RndMeth=Zero
  Output : Outport
  wires:
  In2/1 -> Divide4/2
  In1/1 -> Divide4/1
  Divide4/1 -> Output/1, Display2/1

== system Power_Grid_Fault_Analysis_2016/For Zone 5/Subsystem3 ==
  In1 : Inport
  In2 : Inport  Port=2
  Display2 : Display
      settings: Decimation=2
  Divide4 : Product  Inputs=**  SaturateOnIntegerOverflow=on  RndMeth=Zero
  Output : Outport
  wires:
  In2/1 -> Divide4/2
  In1/1 -> Divide4/1
  Divide4/1 -> Output/1, Display2/1

== system Power_Grid_Fault_Analysis_2016/For Zone 5/Subsystem4 ==
  In1 : Inport
  In2 : Inport  Port=2
  Display2 : Display
      settings: Decimation=2
  Divide4 : Product  Inputs=**  SaturateOnIntegerOverflow=on  RndMeth=Zero
  Output : Outport
  wires:
  Divide4/1 -> Display2/1, Output/1
  In1/1 -> Divide4/1
  In2/1 -> Divide4/2

== system Power_Grid_Fault_Analysis_2016/For Zone 5/Subsystem5 ==
  In1 : Inport
  In2 : Inport  Port=2
  Display2 : Display
      settings: Decimation=2
  Divide4 : Product  Inputs=**  SaturateOnIntegerOverflow=on  RndMeth=Zero
  Output : Outport
  wires:
  In2/1 -> Divide4/2
  In1/1 -> Divide4/1
  Divide4/1 -> Output/1, Display2/1

== system Power_Grid_Fault_Analysis_2016/For Zone 5/Subsystem6 ==
  In1 : Inport
  In2 : Inport  Port=2
  Display2 : Display
      settings: Decimation=2
  Divide4 : Product  Inputs=**  SaturateOnIntegerOverflow=on  RndMeth=Zero
  Output : Outport
  wires:
  Divide4/1 -> Display2/1, Output/1
  In1/1 -> Divide4/1
  In2/1 -> Divide4/2

== system Power_Grid_Fault_Analysis_2016/For Zone 5/Subsystem7 ==
  In1 : Inport
  In2 : Inport  Port=2
  Display2 : Display
      settings: Decimation=2
  Divide4 : Product  Inputs=**  SaturateOnIntegerOverflow=on  RndMeth=Zero
  Output : Outport
  wires:
  In2/1 -> Divide4/2
  In1/1 -> Divide4/1
  Divide4/1 -> Output/1, Display2/1

== system Power_Grid_Fault_Analysis_2016/Relay /AC Time Overcurrent Relay2 ==
  I : Inport
  Clock : Clock
  Irms : powerlib_meascontrol/Measurements/RMS  TrueRMS=on  Freq=Freq  RMSInit=RMSInit  Ts=0
  Relational Operator : RelationalOperator  Operator=<=  OutDataTypeStr=boolean
  Time Relay Function : MATLAB Function  TreatAsAtomicUnit=on
  C.B : Outport
  OT : Outport  Port=2
  wires:
  Clock/1 -> Relational Operator/1, Time Relay Function/1(clk)
  Irms/1 -> Time Relay Function/2(Irms)
  Time Relay Function/1(TT) -> Relational Operator/2
  Time Relay Function/2(OT) -> OT/1
  Relational Operator/1 -> C.B/1
  I/1 -> Irms/1

== system Power_Grid_Fault_Analysis_2016/Relay /Output1 ==
  Signal : Inport
  Demux : Demux  Outputs=3
  Scope : Scope  NumInputPorts=3
  wires:
  Demux/3 -> Scope/3
  Demux/1 -> Scope/1
  Demux/2 -> Scope/2
  Signal/1 -> Demux/1

== system Power_Grid_Fault_Analysis_2016/Relay /Subsystem ==
  In1 : Inport
  Constant : Constant  Value=5
  Data Type Conversion : DataTypeConversion  OutDataTypeStr=boolean
  Display1 : Display
  NOT : Logic  Operator=NOT  IconShape=distinctive  AllPortsSameDT=off  OutDataTypeStr=boolean
  Sum : Sum  Inputs=|+-
  To Workspace : ToWorkspace  VariableName=G_F_1  SaveFormat=Timeseries  SampleTime=-1
  wires:
  Data Type Conversion/1 -> NOT/1
  Constant/1 -> Sum/2
  Sum/1 -> Data Type Conversion/1
  In1/1 -> To Workspace/1, Sum/1
  NOT/1 -> Display1/1

== system Power_Grid_Fault_Analysis_2016/Relay 1/AC Time Overcurrent Relay2 ==
  I : Inport
  Clock : Clock
  Irms : powerlib_meascontrol/Measurements/RMS  TrueRMS=on  Freq=Freq  RMSInit=RMSInit  Ts=0
  Relational Operator : RelationalOperator  Operator=<=  OutDataTypeStr=boolean
  Time Relay Function : MATLAB Function  TreatAsAtomicUnit=on
  C.B : Outport
  OT : Outport  Port=2
  wires:
  Clock/1 -> Relational Operator/1, Time Relay Function/1(clk)
  Irms/1 -> Time Relay Function/2(Irms)
  Time Relay Function/1(TT) -> Relational Operator/2
  Time Relay Function/2(OT) -> OT/1
  Relational Operator/1 -> C.B/1
  I/1 -> Irms/1

== system Power_Grid_Fault_Analysis_2016/Relay 1/Output1 ==
  Signal : Inport
  Demux : Demux  Outputs=3
  Scope : Scope  NumInputPorts=3
  wires:
  Demux/3 -> Scope/3
  Demux/1 -> Scope/1
  Demux/2 -> Scope/2
  Signal/1 -> Demux/1

== system Power_Grid_Fault_Analysis_2016/Relay 1/Subsystem ==
  In1 : Inport
  Constant : Constant  Value=5
  Data Type Conversion : DataTypeConversion  OutDataTypeStr=boolean
  Display1 : Display
  NOT : Logic  Operator=NOT  IconShape=distinctive  AllPortsSameDT=off  OutDataTypeStr=boolean
  Sum : Sum  Inputs=|+-
  To Workspace : ToWorkspace  VariableName=G_F_R_1  SaveFormat=Timeseries  SampleTime=-1
  wires:
  Data Type Conversion/1 -> NOT/1
  Constant/1 -> Sum/2
  Sum/1 -> Data Type Conversion/1
  In1/1 -> To Workspace/1, Sum/1
  NOT/1 -> Display1/1

== system Power_Grid_Fault_Analysis_2016/Relay 2/AC Time Overcurrent Relay2 ==
  I : Inport
  Clock : Clock
  Irms : powerlib_meascontrol/Measurements/RMS  TrueRMS=on  Freq=Freq  RMSInit=RMSInit  Ts=0
  Relational Operator : RelationalOperator  Operator=<=  OutDataTypeStr=boolean
  Time Relay Function : MATLAB Function  TreatAsAtomicUnit=on
  C.B : Outport
  OT : Outport  Port=2
  wires:
  Clock/1 -> Relational Operator/1, Time Relay Function/1(clk)
  Irms/1 -> Time Relay Function/2(Irms)
  Time Relay Function/1(TT) -> Relational Operator/2
  Time Relay Function/2(OT) -> OT/1
  Relational Operator/1 -> C.B/1
  I/1 -> Irms/1

== system Power_Grid_Fault_Analysis_2016/Relay 2/Output1 ==
  Signal : Inport
  Demux : Demux  Outputs=3
  Scope : Scope  NumInputPorts=3
  wires:
  Demux/3 -> Scope/3
  Demux/1 -> Scope/1
  Demux/2 -> Scope/2
  Signal/1 -> Demux/1

== system Power_Grid_Fault_Analysis_2016/Relay 2/Subsystem ==
  In1 : Inport
  Constant : Constant  Value=5
  Data Type Conversion : DataTypeConversion  OutDataTypeStr=boolean
  Display1 : Display
  NOT : Logic  Operator=NOT  IconShape=distinctive  AllPortsSameDT=off  OutDataTypeStr=boolean
  Sum : Sum  Inputs=|+-
  To Workspace : ToWorkspace  VariableName=G_F_R_2  SaveFormat=Timeseries  SampleTime=-1
  wires:
  Data Type Conversion/1 -> NOT/1
  Constant/1 -> Sum/2
  Sum/1 -> Data Type Conversion/1
  In1/1 -> To Workspace/1, Sum/1
  NOT/1 -> Display1/1

== system Power_Grid_Fault_Analysis_2016/Relay 3/AC Time Overcurrent Relay2 ==
  I : Inport
  Clock : Clock
  Irms : powerlib_meascontrol/Measurements/RMS  TrueRMS=on  Freq=Freq  RMSInit=RMSInit  Ts=0
  Relational Operator : RelationalOperator  Operator=<=  OutDataTypeStr=boolean
  Time Relay Function : MATLAB Function  TreatAsAtomicUnit=on
  C.B : Outport
  OT : Outport  Port=2
  wires:
  Clock/1 -> Relational Operator/1, Time Relay Function/1(clk)
  Irms/1 -> Time Relay Function/2(Irms)
  Time Relay Function/1(TT) -> Relational Operator/2
  Time Relay Function/2(OT) -> OT/1
  Relational Operator/1 -> C.B/1
  I/1 -> Irms/1

== system Power_Grid_Fault_Analysis_2016/Relay 3/Output1 ==
  Signal : Inport
  Demux : Demux  Outputs=3
  Scope : Scope  NumInputPorts=3
  wires:
  Demux/3 -> Scope/3
  Demux/1 -> Scope/1
  Demux/2 -> Scope/2
  Signal/1 -> Demux/1

== system Power_Grid_Fault_Analysis_2016/Relay 3/Subsystem ==
  In1 : Inport
  Constant : Constant  Value=5
  Data Type Conversion : DataTypeConversion  OutDataTypeStr=boolean
  Display1 : Display
  NOT : Logic  Operator=NOT  IconShape=distinctive  AllPortsSameDT=off  OutDataTypeStr=boolean
  Sum : Sum  Inputs=|+-
  To Workspace : ToWorkspace  VariableName=G_F_R_3  SaveFormat=Timeseries  SampleTime=-1
  wires:
  Data Type Conversion/1 -> NOT/1
  Constant/1 -> Sum/2
  Sum/1 -> Data Type Conversion/1
  In1/1 -> To Workspace/1, Sum/1
  NOT/1 -> Display1/1

== system Power_Grid_Fault_Analysis_2016/Relay 4/AC Time Overcurrent Relay2 ==
  I : Inport
  Clock : Clock
  Irms : powerlib_meascontrol/Measurements/RMS  TrueRMS=on  Freq=Freq  RMSInit=RMSInit  Ts=0
  Relational Operator : RelationalOperator  Operator=<=  OutDataTypeStr=boolean
  Time Relay Function : MATLAB Function  TreatAsAtomicUnit=on
  C.B : Outport
  OT : Outport  Port=2
  wires:
  Clock/1 -> Relational Operator/1, Time Relay Function/1(clk)
  Irms/1 -> Time Relay Function/2(Irms)
  Time Relay Function/1(TT) -> Relational Operator/2
  Time Relay Function/2(OT) -> OT/1
  Relational Operator/1 -> C.B/1
  I/1 -> Irms/1

== system Power_Grid_Fault_Analysis_2016/Relay 4/Output1 ==
  Signal : Inport
  Demux : Demux  Outputs=3
  Scope : Scope  NumInputPorts=3
  wires:
  Demux/3 -> Scope/3
  Demux/1 -> Scope/1
  Demux/2 -> Scope/2
  Signal/1 -> Demux/1

== system Power_Grid_Fault_Analysis_2016/Relay 4/Subsystem ==
  In1 : Inport
  Constant : Constant  Value=5
  Data Type Conversion : DataTypeConversion  OutDataTypeStr=boolean
  Display1 : Display
  NOT : Logic  Operator=NOT  IconShape=distinctive  AllPortsSameDT=off  OutDataTypeStr=boolean
  Sum : Sum  Inputs=|+-
  To Workspace : ToWorkspace  VariableName=G_F_R_4  SaveFormat=Timeseries  SampleTime=-1
  wires:
  Data Type Conversion/1 -> NOT/1
  Constant/1 -> Sum/2
  Sum/1 -> Data Type Conversion/1
  In1/1 -> To Workspace/1, Sum/1
  NOT/1 -> Display1/1

== matlab function Power_Grid_Fault_Analysis_2016/Relay 1/AC Time Overcurrent Relay2/Time Relay Function ==
  settings: updateMethod=DISCRETE
  data: TT output; clk input; Irms input; CTpri parameter; CTsec parameter; PS parameter; OT output; TMS parameter; k parameter; alpha parameter; B parameter; TDS parameter
function [TT, OT] = fcn(clk,Irms,CTpri,CTsec,PS,TMS,k,alpha,B,TDS)

persistent RelayState TripTime OperatingTime PickupTime

if isempty(RelayState)
    RelayState = 0;
    TripTime = inf;
    OperatingTime = inf;
    PickupTime = 0;
end

CT = max(Irms/(CTpri/CTsec));
Pickup = (PS*0.25)*CTsec;

if (RelayState == 0)&&(CT > Pickup)
    PickupTime = clk;
    RelayState = 1;
end

if (RelayState == 1)&&(clk>(PickupTime+0.02)) % Wait for 20ms fault current rise time
    if k == 0
        OperatingTime = TDS;
    else
        PMS = CT/Pickup;                          % Calculate Plug Multiplier Setting
        OperatingTime = ((k/((PMS^alpha)-1))+B)*(TMS*0.05); % Determine Definite Inverse Minimum Time
    end
    TripTime = PickupTime + OperatingTime;
    RelayState = 2;
end

TT = TripTime;
OT = OperatingTime;

== matlab function Power_Grid_Fault_Analysis_2016/Relay 2/AC Time Overcurrent Relay2/Time Relay Function ==
  settings: updateMethod=DISCRETE
  data: TT output; clk input; Irms input; CTpri parameter; CTsec parameter; PS parameter; OT output; TMS parameter; k parameter; alpha parameter; B parameter; TDS parameter
function [TT, OT] = fcn(clk,Irms,CTpri,CTsec,PS,TMS,k,alpha,B,TDS)

persistent RelayState TripTime OperatingTime PickupTime

if isempty(RelayState)
    RelayState = 0;
    TripTime = inf;
    OperatingTime = inf;
    PickupTime = 0;
end

CT = max(Irms/(CTpri/CTsec));
Pickup = (PS*0.25)*CTsec;

if (RelayState == 0)&&(CT > Pickup)
    PickupTime = clk;
    RelayState = 1;
end

if (RelayState == 1)&&(clk>(PickupTime+0.02)) % Wait for 20ms fault current rise time
    if k == 0
        OperatingTime = TDS;
    else
        PMS = CT/Pickup;                          % Calculate Plug Multiplier Setting
        OperatingTime = ((k/((PMS^alpha)-1))+B)*(TMS*0.05); % Determine Definite Inverse Minimum Time
    end
    TripTime = PickupTime + OperatingTime;
    RelayState = 2;
end

TT = TripTime;
OT = OperatingTime;

== matlab function Power_Grid_Fault_Analysis_2016/Relay /AC Time Overcurrent Relay2/Time Relay Function ==
  settings: updateMethod=DISCRETE
  data: TT output; clk input; Irms input; CTpri parameter; CTsec parameter; PS parameter; OT output; TMS parameter; k parameter; alpha parameter; B parameter; TDS parameter
function [TT, OT] = fcn(clk,Irms,CTpri,CTsec,PS,TMS,k,alpha,B,TDS)

persistent RelayState TripTime OperatingTime PickupTime

if isempty(RelayState)
    RelayState = 0;
    TripTime = inf;
    OperatingTime = inf;
    PickupTime = 0;
end

CT = max(Irms/(CTpri/CTsec));
Pickup = (PS*0.25)*CTsec;

if (RelayState == 0)&&(CT > Pickup)
    PickupTime = clk;
    RelayState = 1;
end

if (RelayState == 1)&&(clk>(PickupTime+0.02)) % Wait for 20ms fault current rise time
    if k == 0
        OperatingTime = TDS;
    else
        PMS = CT/Pickup;                          % Calculate Plug Multiplier Setting
        OperatingTime = ((k/((PMS^alpha)-1))+B)*(TMS*0.05); % Determine Definite Inverse Minimum Time
    end
    TripTime = PickupTime + OperatingTime;
    RelayState = 2;
end

TT = TripTime;
OT = OperatingTime;

== matlab function Power_Grid_Fault_Analysis_2016/Relay 3/AC Time Overcurrent Relay2/Time Relay Function ==
  settings: updateMethod=DISCRETE
  data: TT output; clk input; Irms input; CTpri parameter; CTsec parameter; PS parameter; OT output; TMS parameter; k parameter; alpha parameter; B parameter; TDS parameter
function [TT, OT] = fcn(clk,Irms,CTpri,CTsec,PS,TMS,k,alpha,B,TDS)

persistent RelayState TripTime OperatingTime PickupTime

if isempty(RelayState)
    RelayState = 0;
    TripTime = inf;
    OperatingTime = inf;
    PickupTime = 0;
end

CT = max(Irms/(CTpri/CTsec));
Pickup = (PS*0.25)*CTsec;

if (RelayState == 0)&&(CT > Pickup)
    PickupTime = clk;
    RelayState = 1;
end

if (RelayState == 1)&&(clk>(PickupTime+0.02)) % Wait for 20ms fault current rise time
    if k == 0
        OperatingTime = TDS;
    else
        PMS = CT/Pickup;                          % Calculate Plug Multiplier Setting
        OperatingTime = ((k/((PMS^alpha)-1))+B)*(TMS*0.05); % Determine Definite Inverse Minimum Time
    end
    TripTime = PickupTime + OperatingTime;
    RelayState = 2;
end

TT = TripTime;
OT = OperatingTime;

== matlab function Power_Grid_Fault_Analysis_2016/Relay 4/AC Time Overcurrent Relay2/Time Relay Function ==
  settings: updateMethod=DISCRETE
  data: TT output; clk input; Irms input; CTpri parameter; CTsec parameter; PS parameter; OT output; TMS parameter; k parameter; alpha parameter; B parameter; TDS parameter
function [TT, OT] = fcn(clk,Irms,CTpri,CTsec,PS,TMS,k,alpha,B,TDS)

persistent RelayState TripTime OperatingTime PickupTime

if isempty(RelayState)
    RelayState = 0;
    TripTime = inf;
    OperatingTime = inf;
    PickupTime = 0;
end

CT = max(Irms/(CTpri/CTsec));
Pickup = (PS*0.25)*CTsec;

if (RelayState == 0)&&(CT > Pickup)
    PickupTime = clk;
    RelayState = 1;
end

if (RelayState == 1)&&(clk>(PickupTime+0.02)) % Wait for 20ms fault current rise time
    if k == 0
        OperatingTime = TDS;
    else
        PMS = CT/Pickup;                          % Calculate Plug Multiplier Setting
        OperatingTime = ((k/((PMS^alpha)-1))+B)*(TMS*0.05); % Determine Definite Inverse Minimum Time
    end
    TripTime = PickupTime + OperatingTime;
    RelayState = 2;
end

TT = TripTime;
OT = OperatingTime;
